simulink model "reaction_pendulum_MPC_swing_test"  (R2023b)
settings: Solver=FixedStepDiscrete  StartTime=0.0  StopTime=20  FixedStep=h  RelTol=1e-3  EnableMultiTasking=on
PreLoadFcn:
  | warning('off','MATLAB:dispatcher:InexactMatch');
InitFcn:
  | startup_sequence
StartFcn:
  | startup_sequence
model workspace (MAT data in the model file):
  square_freq = 0.5
values from neighbouring files (symbols this model uses):
  F = A22-L*A12    [Reduced_observer.m]
  G = A21-L*A11+F*L    [Reduced_observer.m]
  H = B2-L*B1    [Reduced_observer.m]
  K_LQR = lqr(A,B,Q,R)    [LQR_gain.m]
  L = 10    [LQR_gain.m]    (also in Reduced_observer.m = place(A22',A12',pole)')
  linearization_point = [0;0;0]    [startup_sequence.m]
  lp_deviation = [pi/9;0;0]    [startup_sequence.m]
undefined symbols (not defined in the file or in its folder): DiscIntNeverNeededParam, H_nlobs
libraries: mpclib x2
settings Model: ExtModeTrigDuration=100000  Creator=user  LastModifiedBy=india
settings DataIOCC: SaveFormat=Array  SignalLoggingSaveFormat=ModelDataLogs  SaveOutput=off  SignalLogging=off  DSMLogging=off  SaveTime=off  ReturnWorkspaceOutputs=off
settings OptimizationCC: ExpressionDepthLimit=2147483647  LifeSpan=inf
settings DebuggingCC: UnderspecifiedInitializationDetection=Classic  MergeDetectMultiDrivingBlocksExec=none  SolverPrmCheckMsg=warning  FcnCallInpInsideContextMsg=warning  UnconnectedInputMsg=warning  UnconnectedOutputMsg=warning  UnconnectedLineMsg=warning  StateNameClashWarn=warning  SFUnexpectedBacktrackingDiag=warning  SFNoUnconditionalDefaultTransitionDiag=warning  SFExecutionAtInitializationDiag=none  ArithmeticOperatorsInVariantConditions=warning
settings HardwareCC: ProdBitPerPointer=32  ProdBitPerSizeT=32  ProdBitPerPtrDiffT=32  ProdLargestAtomicFloat=None  ProdIntDivRoundTo=Undefined  ProdEndianess=Unspecified  ProdWordSize=32  ProdHWDeviceType=32-bit Generic
settings ModelReferenceCC: EnableRefExpFcnMdlSchedulingChecks=on  PropagateSignalLabelsOutOfModel=off
settings SFSimCC: SimUseLocalCustomCode=off  CustomCodeUndefinedFunction=UseInterfaceOnly
settings RTWCC: Description=rpend RTDAC/USB2 (Visual C/C++)  SystemTargetFile=rtcon_rpend_usb2.tlc  TemplateMakefile=rtcon_rpend_vc_usb2_x64.tmf  RTWUseLocalCustomCode=off  DLArmComputeVersion=19.05
settings CodeAppCC: StateflowObjectComments=on
settings STFCustomTargetCC: TargetLangStandard=C89/C90 (ANSI)  ModelReferenceCompliant=off  CombineOutputUpdateFcns=on  MatFileLogging=on  SystemTargetFile=rtcon_rpend_usb2.tlc
settings GRTTargetCC: TargetLangStandard=C89/C90 (ANSI)  ModelReferenceCompliant=off  ParMdlRefBuildCompliant=off  CompOptLevelCompliant=off  ConcurrentExecutionCompliant=off  CPPClassGenCompliant=off  UseToolchainInfoCompliant=off  ExtMode=on  ExtModeMexFile=rtcon_ext_comm
settings ConfigComp: CovMetricSettings=dw  CovSaveCumulativeToWorkspaceVar=on  CovSaveSingleToWorkspaceVar=on  CovExternalEMLEnable=off  CovSFcnEnable=off

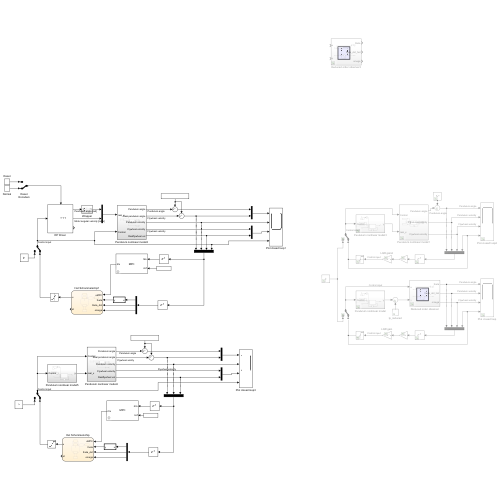
[thumbnail: Simulink's stored preview of the top-level diagram]
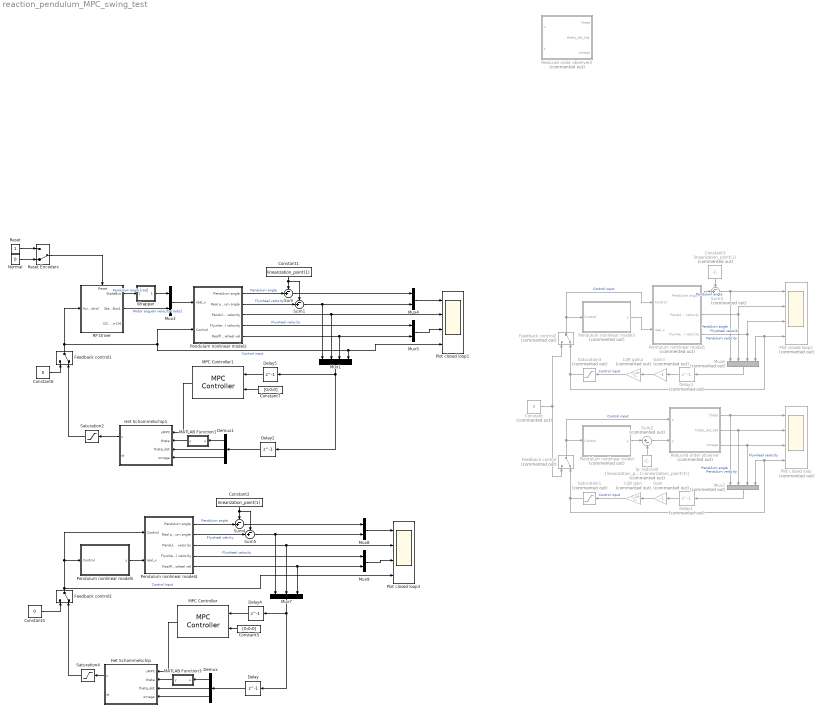
== system reaction_pendulum_MPC_swing_test ==
  Constant : Constant  Commented=on  Value=0
  Constant1 : Constant  Value=linearization_point(1)
  Constant2 : Constant  Value=linearization_point(1)
  Constant3 : Constant  Commented=on  Value=linearization_point(1)
  Constant4 : Constant  Value=0
  Constant5 : Constant  Value=[0;0;0]
  Constant6 : Constant  Value=0
  Constant7 : Constant  Value=[0;0;0]
  Delay{,2,4..5} (4 alike) : Delay  DelayLength=1
  Delay1 : Delay  Commented=on  DelayLength=1
  Delay3 : Delay  Commented=on  DelayLength=1
  Demux : Demux  Outputs=3
  Demux1 : Demux  Outputs=3
  Feedback control : ManualSwitch  Commented=on  CurrentSetting=0
  Feedback control1 : ManualSwitch  CurrentSetting=0
  Feedback control2 : ManualSwitch  Commented=on  CurrentSetting=0
  Feedback control3 : ManualSwitch  CurrentSetting=0
  Gain : Gain  Commented=on  Gain=-1
  Gain3 : Gain  Commented=on  Gain=-1
  Het Schommelschip : Stateflow chart  TreatAsAtomicUnit=on
      settings: PortSchema="{\"entries\":[{\"content\":{\"sides\":[{\"content\":{\"connectorIds\":[\"In3\",\"In1\",\"In2\",\"In4\"]},\"type\":\"ConnectorPlacement.EquallySpacedRectSide\",\"uuid\":\"5e0e74da-86d0-4b0f-97b8-22d473cf7e44\"},{\"content\":{\"connectorIds\":[\"Out1\",\"Out2\"],\"side\":\"RIGHT\"},\"type\":\"ConnectorPlacement.EquallySpacedRectSide\",\"uuid\":\"714d43ea-69d2-420e-91fb-73cc0bbad146\"},{\"content\":{\"side\":\"TOP\"},\"type\":\"ConnectorPlacement.EquallySpacedRectSide\",\"uuid\":\"53d3d334-5a38-461d-a9d2-49aa371a08e3\"}]},\"type\":\"ConnectorPlacement.EquallySpacedConnector\",\"uuid\":\"bed2510c-5cc6-4076-81b8-1d254a2b08c8\"}],\"packageUris\":[\"http://schema.mathworks.com/mf0/Connector/R2020b\"],\"version\":\"1.0\"}"
  Het Schommelschip1 : Stateflow chart  TreatAsAtomicUnit=on
      settings: PortSchema="{\"entries\":[{\"content\":{\"sides\":[{\"content\":{\"connectorIds\":[\"In3\",\"In1\",\"In2\",\"In4\"]},\"type\":\"ConnectorPlacement.EquallySpacedRectSide\",\"uuid\":\"5e0e74da-86d0-4b0f-97b8-22d473cf7e44\"},{\"content\":{\"connectorIds\":[\"Out1\",\"Out2\"],\"side\":\"RIGHT\"},\"type\":\"ConnectorPlacement.EquallySpacedRectSide\",\"uuid\":\"714d43ea-69d2-420e-91fb-73cc0bbad146\"},{\"content\":{\"side\":\"TOP\"},\"type\":\"ConnectorPlacement.EquallySpacedRectSide\",\"uuid\":\"53d3d334-5a38-461d-a9d2-49aa371a08e3\"}]},\"type\":\"ConnectorPlacement.EquallySpacedConnector\",\"uuid\":\"bed2510c-5cc6-4076-81b8-1d254a2b08c8\"}],\"packageUris\":[\"http://schema.mathworks.com/mf0/Connector/R2020b\"],\"version\":\"1.0\"}"
  LQR gain : Gain  Commented=on  Gain=K_LQR  Multiplication=Matrix(K*u)
  LQR gain2 : Gain  Commented=on  Gain=K_LQR  Multiplication=Matrix(K*u)
  MATLAB Function1 : MATLAB Function  TreatAsAtomicUnit=on
  MATLAB Function3 : MATLAB Function  TreatAsAtomicUnit=on
  MPC Controller : mpclib/MPC Controller  SCDEnableBlockLinearizationSpecification=on  mpcobj=mpc_controller  is_multiple=0  enable_value=0  return_u0=off  updateMPCinCallerWorkspace=on  md_inport=off  mv_inport=off  uref_inport=off  return_cost=off  return_mvseq=off  return_qpstatus=off  return_xseq=off  return_state=off  return_ovseq=off  state_inport=off  umin_inport=off  umax_inport=off  ymin_inport=off  ymax_inport=off  cc_inport=off  ywt_inport=off  uwt_inport=off  duwt_inport=off  rhoeps_inport=off  pm_inport=off  MaximumP=10  HorizonChoice=FixedHorizon  n_ts=0.01  n_p=20  n_mv=1  n_md=0  n_ud=0  n_mo=3  n_uo=0  BlockDataType=double  SampleTimeInherited=off  switch_inport=off
  MPC Controller1 : mpclib/MPC Controller  SCDEnableBlockLinearizationSpecification=on  mpcobj=mpc_controller  is_multiple=0  enable_value=0  return_u0=off  updateMPCinCallerWorkspace=on  md_inport=off  mv_inport=off  uref_inport=off  return_cost=off  return_mvseq=off  return_qpstatus=off  return_xseq=off  return_state=off  return_ovseq=off  state_inport=off  umin_inport=off  umax_inport=off  ymin_inport=off  ymax_inport=off  cc_inport=off  ywt_inport=off  uwt_inport=off  duwt_inport=off  rhoeps_inport=off  pm_inport=off  MaximumP=10  HorizonChoice=FixedHorizon  n_ts=0.01  n_p=20  n_mv=1  n_md=0  n_ud=0  n_mo=3  n_uo=0  BlockDataType=double  SampleTimeInherited=off  switch_inport=off
  Mux1 : Mux
  Mux2 : Mux  Commented=on
  Mux{3..5,8..9} (5 alike) : Mux  Inputs=2
  Mux6 : Mux  Commented=on
  Mux7 : Mux  Inputs=3
  Normal : Constant  Value=0
  Pendulum nonlinear model : Subsystem  Commented=on
  Pendulum nonlinear model1 : Subsystem  Commented=on
  Pendulum nonlinear model2 : Subsystem
  Pendulum nonlinear model3 : Subsystem  Commented=on
  Pendulum nonlinear model4 : Subsystem
  Pendulum nonlinear model5 : Subsystem
  Plot closed loop : Scope  Commented=on  NumInputPorts=4
  Plot closed loop1 : Scope  NumInputPorts=4
  Plot closed loop2 : Scope  Commented=on  NumInputPorts=4
  Plot closed loop3 : Scope  NumInputPorts=4
  RP Driver : Subsystem
      settings: PortSchema="{\"entries\":[{\"content\":{\"sides\":[{\"content\":{\"connectorIds\":[\"In1\"]},\"type\":\"ConnectorPlacement.EquallySpacedRectSide\",\"uuid\":\"28df0a7f-6242-4d39-ac1c-ff3ee0c6a4e1\"},{\"content\":{\"connectorIds\":[\"Out1\",\"Out2\",\"Out3\"],\"side\":\"RIGHT\"},\"type\":\"ConnectorPlacement.EquallySpacedRectSide\",\"uuid\":\"435de4ce-8687-493c-bad7-12ebb99ee6db\"},{\"content\":{\"connectorIds\":[\"In2\"],\"side\":\"TOP\"},\"type\":\"ConnectorPlacement.EquallySpacedRectSide\",\"uuid\":\"946ce8c1-4b6f-49e8-9b13-de0bfa90dc27\"},{\"content\":{\"side\":\"BOTTOM\"},\"type\":\"ConnectorPlacement.EquallySpacedRectSide\",\"uuid\":\"2521f2e0-71e2-448f-85b3-c4d5eb7ca065\"}]},\"type\":\"ConnectorPlacement.EquallySpacedConnector\",\"uuid\":\"0b989423-35e3-4087-b06d-cef0c97f9c21\"}],\"packageUris\":[\"http://schema.mathworks.com/mf0/Connector/R2020b\"],\"version\":\"1.0\"}"
      mask Display: image(imread('rwp.JPG'))
  Reduced order observer : Subsystem  Commented=on
  Reduced order observer2 : Subsystem  Commented=on
  Reset : Constant
  Reset Encoders : ManualSwitch  CurrentSetting=0
  Saturation1 : Saturate  Commented=on  UpperLimit=1  LowerLimit=-1
  Saturation2 : Saturate  UpperLimit=1  LowerLimit=-1
  Saturation3 : Saturate  Commented=on  UpperLimit=1  LowerLimit=-1
  Saturation4 : Saturate  UpperLimit=1  LowerLimit=-1
  Sum{,1,4..5} (4 alike) : Sum  Inputs=-+|
  Sum2 : Sum  Commented=on  Inputs=|+-
  Sum3 : Sum  Commented=on  Inputs=-+|
  Wrapper : Subsystem
  lp_reduced : Constant  Commented=on  Value=[linearization_point(1);linearization_point(3)]
  wires:
  Normal/1 -> Reset Encoders/2
  Reset/1 -> Reset Encoders/1
  Reset Encoders/1 -> RP Driver/2(Reset)
  RP Driver/1(StateBus) -> Wrapper/1(In1)  "Pendulum angle [rad]"
  Feedback control/1 -> Reduced order observer/1(u), Pendulum nonlinear model/1(Control)  "Control input"
  LQR gain/1 -> Saturation1/1  "Control input"
  Gain/1 -> LQR gain/1
  Delay1/1 -> Gain/1
  Reduced order observer/2(theta_dot_hat) -> Plot closed loop/2, Mux2/2  "Pendulum velocity"
  Sum2/1 -> Reduced order observer/2(y)
  lp_reduced/1 -> Sum2/2
  Pendulum nonlinear model/1(y) -> Sum2/1
  Reduced order observer/1(theta) -> Plot closed loop/1, Mux2/1  "Pendulum angle"
  Reduced order observer/3(omega) -> Plot closed loop/3, Mux2/3  "Flywheel velocity"
  Mux2/1 -> Delay1/1
  Feedback control1/1 -> Pendulum nonlinear model2/2(Control), Mux1/4, Plot closed loop1/4, RP Driver/1(Azimuth Control)  "Control input"
  Saturation1/1 -> Plot closed loop/4, Mux2/4, Feedback control/2
  Constant1/1 -> Sum1/1, Sum/1
  Wrapper/1(Out1) -> Mux3/1
  Mux4/1 -> Plot closed loop1/1
  Mux5/1 -> Plot closed loop1/3
  Sum1/1 -> Mux4/2, Mux1/1
  Pendulum nonlinear model1/1(Pendulum angle) -> Sum3/2  "Pendulum angle"
  Constant3/1 -> Sum3/1
  Saturation3/1 -> Plot closed loop2/4, Mux6/4, Feedback control2/2
  Pendulum nonlinear model3/1(y) -> Pendulum nonlinear model1/2(real_x)
  Sum3/1 -> Plot closed loop2/1, Mux6/1  "Pendulum angle"
  Gain3/1 -> LQR gain2/1
  Pendulum nonlinear model1/2(Pendulum velocity) -> Plot closed loop2/2, Mux6/2  "Pendulum velocity"
  LQR gain2/1 -> Saturation3/1  "Control input"
  Pendulum nonlinear model1/3(Flywheel velocity) -> Plot closed loop2/3, Mux6/3  "Flywheel velocity"
  Mux6/1 -> Delay3/1
  Delay3/1 -> Gain3/1
  Feedback control2/1 -> Pendulum nonlinear model3/1(Control), Pendulum nonlinear model1/1(Control)  "Control input"
  Constant/1 -> Feedback control/1, Feedback control2/1
  Feedback control3/1 -> Pendulum nonlinear model4/1(Control), Pendulum nonlinear model5/1(Control), Plot closed loop3/4  "Control input"
  Pendulum nonlinear model5/1(y) -> Pendulum nonlinear model4/2(real_x)
  Constant4/1 -> Feedback control3/1
  Constant6/1 -> Feedback control1/1
  RP Driver/2(StateBus1) -> Mux3/2  "Motor angular velocity [rad/s]"
  Sum/1 -> Mux4/1
  Sum4/1 -> Mux8/1
  Pendulum nonlinear model4/4(Flywheel velocity) -> Mux9/1  "Flywheel velocity"
  Pendulum nonlinear model4/5(Realflywheel vel) -> Mux7/3, Mux9/2
  Mux9/1 -> Plot closed loop3/3
  Mux8/1 -> Plot closed loop3/1
  Sum5/1 -> Mux8/2, Mux7/1
  Pendulum nonlinear model4/1(Pendulum angle) -> Sum4/2  "Pendulum angle"
  Constant2/1 -> Sum5/1, Sum4/1
  Mux7/1 -> Delay/1, Delay4/1
  Pendulum nonlinear model4/3(Pendulum velocity) -> Mux7/2, Plot closed loop3/2
  Pendulum nonlinear model4/2(Real pendulum angle) -> Sum5/2  "Flywheel velcity"
  Pendulum nonlinear model2/1(Pendulum angle) -> Sum/2  "Pendulum angle"
  Pendulum nonlinear model2/2(Real pendulum angle) -> Sum1/2  "Flywheel velocity"
  Pendulum nonlinear model2/3(Pendulum velocity) -> Mux1/2, Plot closed loop1/2
  Pendulum nonlinear model2/4(Flywheel velocity) -> Mux5/1  "Flywheel velocity"
  Pendulum nonlinear model2/5(Realflywheel vel) -> Mux5/2, Mux1/3
  Mux3/1 -> Pendulum nonlinear model2/1(real_x)
  Delay4/1 -> MPC Controller/1
  Demux/3 -> Het Schommelschip/4(omega)
  Demux/1 -> MATLAB Function3/1(u)
  MATLAB Function3/1(y) -> Het Schommelschip/1(theta)
  Demux/2 -> Het Schommelschip/2(theta_dot)
  Het Schommelschip/1(u) -> Saturation4/1
  MPC Controller/1 -> Het Schommelschip/3(uMPC)
  Constant5/1 -> MPC Controller/2
  Delay/1 -> Demux/1
  Saturation4/1 -> Feedback control3/2
  Saturation2/1 -> Feedback control1/2
  Demux1/2 -> Het Schommelschip1/2(theta_dot)
  Delay2/1 -> Demux1/1
  Demux1/1 -> MATLAB Function1/1(u)
  Constant7/1 -> MPC Controller1/2
  Demux1/3 -> Het Schommelschip1/4(omega)
  MPC Controller1/1 -> Het Schommelschip1/3(uMPC)
  MATLAB Function1/1(y) -> Het Schommelschip1/1(theta)
  Delay5/1 -> MPC Controller1/1
  Het Schommelschip1/1(u) -> Saturation2/1
  Mux1/1 -> Delay5/1, Delay2/1

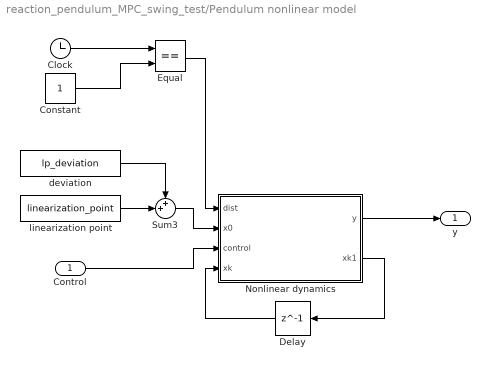
== system reaction_pendulum_MPC_swing_test/Pendulum nonlinear model ==
  Control : Inport
  Clock : Clock
  Constant : Constant
  Delay : Delay  DelayLength=1
  Equal : RelationalOperator  Operator===  OutDataTypeStr=boolean  RndMeth=Simplest  InputSameDT=off
  Nonlinear dynamics : MATLAB Function  TreatAsAtomicUnit=on
  Sum3 : Sum  Inputs=++|
  deviation : Constant  Value=lp_deviation
  linearization point : Constant  Value=linearization_point
  y : Outport
  wires:
  Delay/1 -> Nonlinear dynamics/4(xk)
  Sum3/1 -> Nonlinear dynamics/2(x0)
  Control/1 -> Nonlinear dynamics/3(control)
  Nonlinear dynamics/2(xk1) -> Delay/1
  Nonlinear dynamics/1(y) -> y/1
  deviation/1 -> Sum3/1
  linearization point/1 -> Sum3/2
  Constant/1 -> Equal/2
  Equal/1 -> Nonlinear dynamics/1(dist)
  Clock/1 -> Equal/1

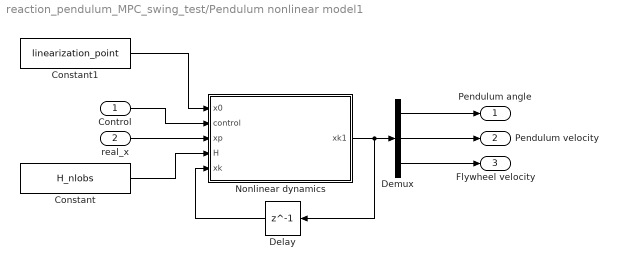
== system reaction_pendulum_MPC_swing_test/Pendulum nonlinear model1 ==
  Control : Inport
  real_x : Inport  Port=2
  Constant : Constant  Value=H_nlobs
  Constant1 : Constant  Value=linearization_point
  Delay : Delay  DelayLength=1
  Demux : Demux  Outputs=3
  Nonlinear dynamics : MATLAB Function  TreatAsAtomicUnit=on
  Pendulum angle : Outport
  Pendulum velocity : Outport  Port=2
  Flywheel velocity : Outport  Port=3
  wires:
  Delay/1 -> Nonlinear dynamics/5(xk)
  Control/1 -> Nonlinear dynamics/2(control)
  Nonlinear dynamics/1(xk1) -> Demux/1, Delay/1
  real_x/1 -> Nonlinear dynamics/3(xp)
  Constant/1 -> Nonlinear dynamics/4(H)
  Constant1/1 -> Nonlinear dynamics/1(x0)
  Demux/2 -> Pendulum velocity/1
  Demux/1 -> Pendulum angle/1
  Demux/3 -> Flywheel velocity/1

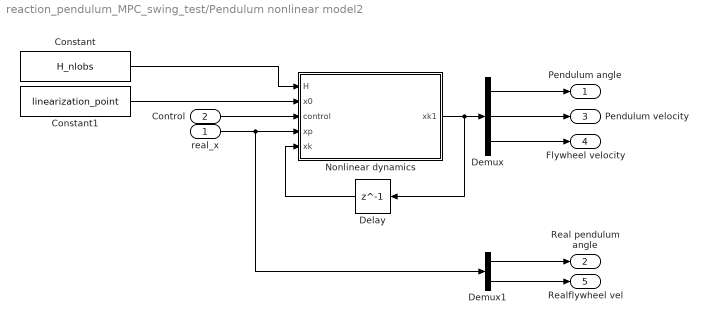
== system reaction_pendulum_MPC_swing_test/Pendulum nonlinear model2 ==
  real_x : Inport
  Control : Inport  Port=2
  Constant : Constant  Value=H_nlobs
  Constant1 : Constant  Value=linearization_point
  Delay : Delay  DelayLength=1
  Demux : Demux  Outputs=3
  Demux1 : Demux  Outputs=2
  Nonlinear dynamics : MATLAB Function  TreatAsAtomicUnit=on
  Pendulum angle : Outport
  Real pendulum angle : Outport  Port=2
  Pendulum velocity : Outport  Port=3
  Flywheel velocity : Outport  Port=4
  Realflywheel vel : Outport  Port=5
  wires:
  Delay/1 -> Nonlinear dynamics/5(xk)
  Control/1 -> Nonlinear dynamics/3(control)
  Nonlinear dynamics/1(xk1) -> Demux/1, Delay/1
  real_x/1 -> Demux1/1, Nonlinear dynamics/4(xp)
  Constant/1 -> Nonlinear dynamics/1(H)
  Constant1/1 -> Nonlinear dynamics/2(x0)
  Demux/2 -> Pendulum velocity/1
  Demux/1 -> Pendulum angle/1
  Demux/3 -> Flywheel velocity/1
  Demux1/1 -> Real pendulum angle/1
  Demux1/2 -> Realflywheel vel/1

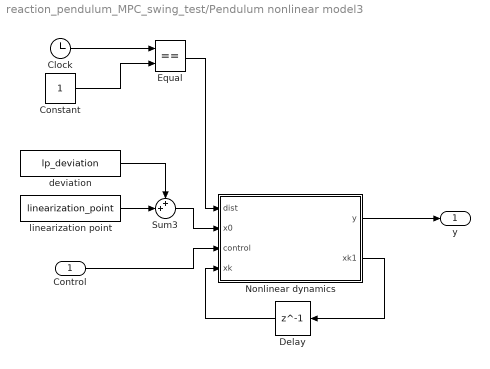
== system reaction_pendulum_MPC_swing_test/Pendulum nonlinear model3 ==
  Control : Inport
  Clock : Clock
  Constant : Constant
  Delay : Delay  DelayLength=1
  Equal : RelationalOperator  Operator===  OutDataTypeStr=boolean  RndMeth=Simplest  InputSameDT=off
  Nonlinear dynamics : MATLAB Function  TreatAsAtomicUnit=on
  Sum3 : Sum  Inputs=++|
  deviation : Constant  Value=lp_deviation
  linearization point : Constant  Value=linearization_point
  y : Outport
  wires:
  Delay/1 -> Nonlinear dynamics/4(xk)
  Sum3/1 -> Nonlinear dynamics/2(x0)
  Control/1 -> Nonlinear dynamics/3(control)
  Nonlinear dynamics/2(xk1) -> Delay/1
  Nonlinear dynamics/1(y) -> y/1
  deviation/1 -> Sum3/1
  linearization point/1 -> Sum3/2
  Clock/1 -> Equal/1
  Constant/1 -> Equal/2
  Equal/1 -> Nonlinear dynamics/1(dist)

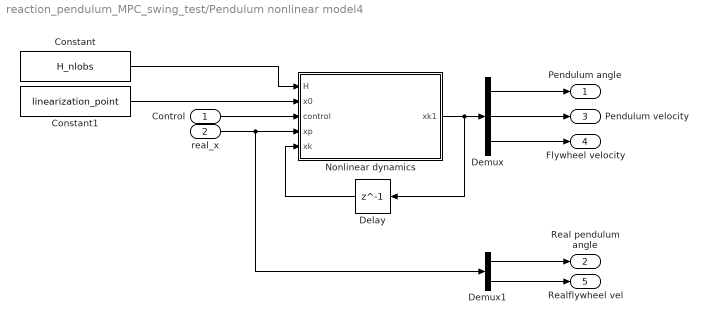
== system reaction_pendulum_MPC_swing_test/Pendulum nonlinear model4 ==
  Control : Inport
  real_x : Inport  Port=2
  Constant : Constant  Value=H_nlobs
  Constant1 : Constant  Value=linearization_point
  Delay : Delay  DelayLength=1
  Demux : Demux  Outputs=3
  Demux1 : Demux  Outputs=2
  Nonlinear dynamics : MATLAB Function  TreatAsAtomicUnit=on
  Pendulum angle : Outport
  Real pendulum angle : Outport  Port=2
  Pendulum velocity : Outport  Port=3
  Flywheel velocity : Outport  Port=4
  Realflywheel vel : Outport  Port=5
  wires:
  Delay/1 -> Nonlinear dynamics/5(xk)
  Control/1 -> Nonlinear dynamics/3(control)
  Nonlinear dynamics/1(xk1) -> Demux/1, Delay/1
  real_x/1 -> Demux1/1, Nonlinear dynamics/4(xp)
  Constant/1 -> Nonlinear dynamics/1(H)
  Constant1/1 -> Nonlinear dynamics/2(x0)
  Demux/2 -> Pendulum velocity/1
  Demux/1 -> Pendulum angle/1
  Demux/3 -> Flywheel velocity/1
  Demux1/1 -> Real pendulum angle/1
  Demux1/2 -> Realflywheel vel/1

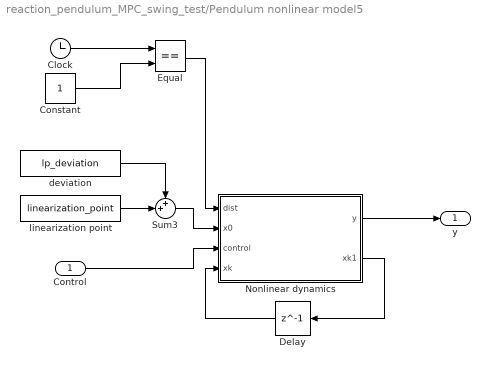
== system reaction_pendulum_MPC_swing_test/Pendulum nonlinear model5 ==
  Control : Inport
  Clock : Clock
  Constant : Constant
  Delay : Delay  DelayLength=1
  Equal : RelationalOperator  Operator===  OutDataTypeStr=boolean  RndMeth=Simplest  InputSameDT=off
  Nonlinear dynamics : MATLAB Function  TreatAsAtomicUnit=on
  Sum3 : Sum  Inputs=++|
  deviation : Constant  Value=lp_deviation
  linearization point : Constant  Value=linearization_point
  y : Outport
  wires:
  Delay/1 -> Nonlinear dynamics/4(xk)
  Sum3/1 -> Nonlinear dynamics/2(x0)
  Control/1 -> Nonlinear dynamics/3(control)
  Nonlinear dynamics/2(xk1) -> Delay/1
  Nonlinear dynamics/1(y) -> y/1
  deviation/1 -> Sum3/1
  linearization point/1 -> Sum3/2
  Clock/1 -> Equal/1
  Constant/1 -> Equal/2
  Equal/1 -> Nonlinear dynamics/1(dist)

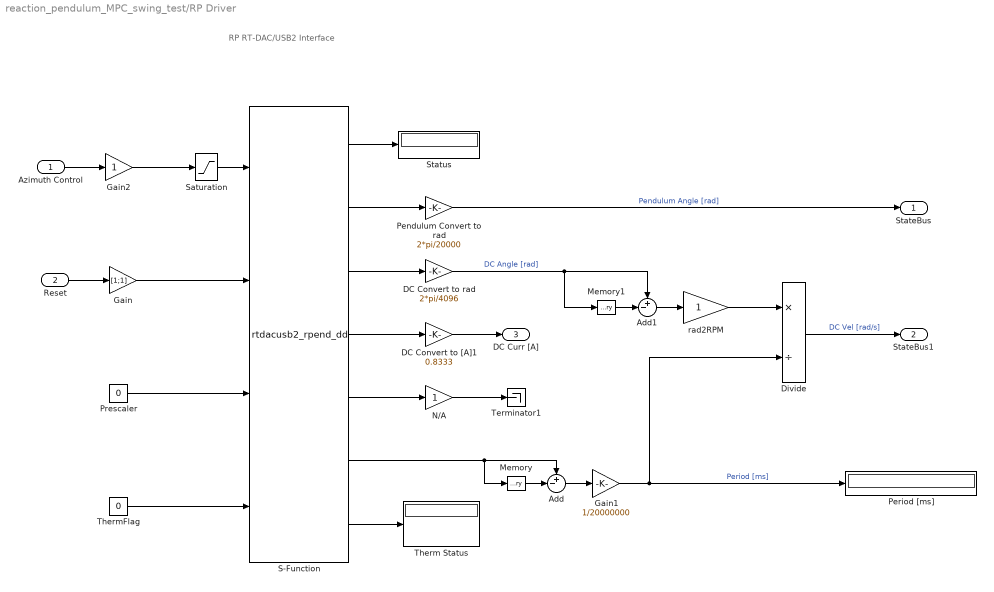
== system reaction_pendulum_MPC_swing_test/RP Driver ==
  note: RP RT-DAC/USB2
      | Interface
  Azimuth Control : Inport
  Reset : Inport  Port=2
  Add : Sum  Inputs=+-|
  Add1 : Sum  Inputs=+-|
  DC Convert to [A]1 : Gain  Gain=0.8333  SaturateOnIntegerOverflow=on  OutDataTypeStr=Inherit: Same as input  ParamDataTypeStr=Inherit: Same as input
  DC Convert to rad : Gain  Gain=2*pi/4096  SaturateOnIntegerOverflow=on  OutDataTypeStr=Inherit: Same as input  ParamDataTypeStr=Inherit: Same as input
  Divide : Product  Inputs=*/
  Gain : Gain  Gain=[1;1]
  Gain1 : Gain  Gain=1/20000000
  Gain2 : Gain
  Memory : Memory
  Memory1 : Memory
  N/A : Gain  SaturateOnIntegerOverflow=on  OutDataTypeStr=Inherit: Same as input  ParamDataTypeStr=Inherit: Same as input
  Pendulum Convert to rad : Gain  Gain=2*pi/20000  SaturateOnIntegerOverflow=on  OutDataTypeStr=Inherit: Same as input  ParamDataTypeStr=Inherit: Same as input
  Period [ms] : Display
  Prescaler : Constant  Value=0
  S-Function : S-Function  FunctionName=rtdacusb2_rpend_dd  Parameters=1, h  SFunctionDeploymentMode=off  EnableBusSupport=off
  Saturation : Saturate  UpperLimit=1  LowerLimit=-1
  Status : Display
  Terminator1 : Terminator
  Therm Status : Display
  ThermFlag : Constant  Value=0
  rad2RPM : Gain  SaturateOnIntegerOverflow=on  OutDataTypeStr=Inherit: Same as input  ParamDataTypeStr=Inherit: Same as input
  StateBus : Outport  VectorParamsAs1DForOutWhenUnconnected=off
  StateBus1 : Outport  Port=2  VectorParamsAs1DForOutWhenUnconnected=off
  DC Curr [A] : Outport  Port=3  VectorParamsAs1DForOutWhenUnconnected=off
  wires:
  S-Function/7 -> Therm Status/1
  S-Function/5 -> N/A/1
  S-Function/4 -> DC Convert to [A]1/1
  ThermFlag/1 -> S-Function/4
  Prescaler/1 -> S-Function/3
  Gain/1 -> S-Function/2
  DC Convert to [A]1/1 -> DC Curr [A]/1
  Divide/1 -> StateBus1/1  "DC Vel [rad/s]"
  rad2RPM/1 -> Divide/1
  Add1/1 -> rad2RPM/1
  Memory1/1 -> Add1/2
  N/A/1 -> Terminator1/1
  S-Function/6 -> Add/1, Memory/1
  Gain2/1 -> Saturation/1
  Gain1/1 -> Period [ms]/1, Divide/2  "Period [ms]"
  Add/1 -> Gain1/1
  Memory/1 -> Add/2
  DC Convert to rad/1 -> Add1/1, Memory1/1  "DC Angle [rad]"
  S-Function/3 -> DC Convert to rad/1
  Pendulum Convert to rad/1 -> StateBus/1  "Pendulum Angle [rad]"
  S-Function/2 -> Pendulum Convert to rad/1
  S-Function/1 -> Status/1
  Saturation/1 -> S-Function/1
  Reset/1 -> Gain/1
  Azimuth Control/1 -> Gain2/1

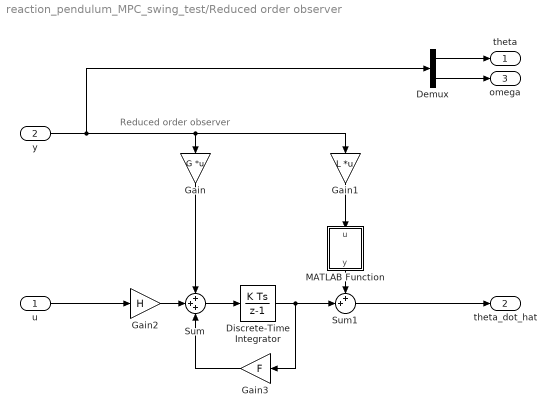
== system reaction_pendulum_MPC_swing_test/Reduced order observer ==
  note: Reduced order observer
  u : Inport
  y : Inport  Port=2
  Demux : Demux  Outputs=2
  Discrete-Time Integrator : DiscreteIntegrator  SampleTime=-1  ICPrevOutput=DiscIntNeverNeededParam  ICPrevScaledInput=DiscIntNeverNeededParam
  Gain : Gain  Gain=G  Multiplication=Matrix(K*u)
  Gain1 : Gain  Gain=L  Multiplication=Matrix(K*u)
  Gain2 : Gain  Gain=H
  Gain3 : Gain  Gain=F
  MATLAB Function : MATLAB Function  TreatAsAtomicUnit=on
  Sum : Sum  Inputs=+++
  Sum1 : Sum  Inputs=++|
  theta : Outport
  theta_dot_hat : Outport  Port=2
  omega : Outport  Port=3
  wires:
  u/1 -> Gain2/1
  Gain2/1 -> Sum/2
  Gain/1 -> Sum/1
  Sum/1 -> Discrete-Time Integrator/1
  Discrete-Time Integrator/1 -> Gain3/1, Sum1/2
  Gain3/1 -> Sum/3
  Sum1/1 -> theta_dot_hat/1
  y/1 -> Gain1/1, Gain/1, Demux/1
  Demux/1 -> theta/1
  Demux/2 -> omega/1
  Gain1/1 -> MATLAB Function/1(u)
  MATLAB Function/1(y) -> Sum1/1

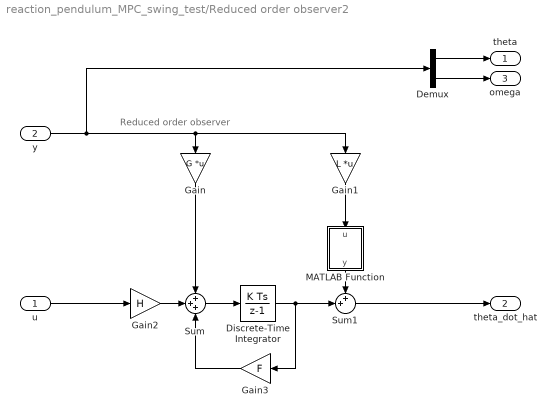
== system reaction_pendulum_MPC_swing_test/Reduced order observer2 ==
  note: Reduced order observer
  u : Inport
  y : Inport  Port=2
  Demux : Demux  Outputs=2
  Discrete-Time Integrator : DiscreteIntegrator  SampleTime=-1  ICPrevOutput=DiscIntNeverNeededParam  ICPrevScaledInput=DiscIntNeverNeededParam
  Gain : Gain  Gain=G  Multiplication=Matrix(K*u)
  Gain1 : Gain  Gain=L  Multiplication=Matrix(K*u)
  Gain2 : Gain  Gain=H
  Gain3 : Gain  Gain=F
  MATLAB Function : MATLAB Function  TreatAsAtomicUnit=on
  Sum : Sum  Inputs=+++
  Sum1 : Sum  Inputs=++|
  theta : Outport
  theta_dot_hat : Outport  Port=2
  omega : Outport  Port=3
  wires:
  u/1 -> Gain2/1
  Gain2/1 -> Sum/2
  Gain/1 -> Sum/1
  Sum/1 -> Discrete-Time Integrator/1
  Discrete-Time Integrator/1 -> Gain3/1, Sum1/2
  Gain3/1 -> Sum/3
  Sum1/1 -> theta_dot_hat/1
  y/1 -> Gain1/1, Gain/1, Demux/1
  Demux/1 -> theta/1
  Demux/2 -> omega/1
  Gain1/1 -> MATLAB Function/1(u)
  MATLAB Function/1(y) -> Sum1/1

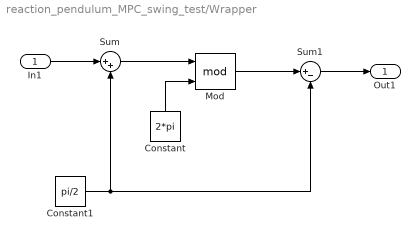
== system reaction_pendulum_MPC_swing_test/Wrapper ==
  In1 : Inport
  Constant : Constant  Value=2*pi
  Constant1 : Constant  Value=pi/2
  Mod : Math  Operator=mod
  Sum : Sum  Inputs=|++
  Sum1 : Sum  Inputs=|+-
  Out1 : Outport
  wires:
  Constant/1 -> Mod/2
  Mod/1 -> Sum1/1
  Sum1/1 -> Out1/1
  In1/1 -> Sum/1
  Sum/1 -> Mod/1
  Constant1/1 -> Sum1/2, Sum/2

== matlab function reaction_pendulum_MPC_swing_test/Reduced order observer2/MATLAB Function ==
  data: u input; y output
function y = fcn(u)
    persistent obs_init
    y=u;
    if isempty(obs_init)
        y=0;
        obs_init = true;
    end
end

== matlab function reaction_pendulum_MPC_swing_test/Pendulum nonlinear model3/Nonlinear dynamics ==
  data: dist input; x0 input; y output; control input; xk input size=[3,1]; xk1 output size=[3,1]; h parameter
function [y, xk1] = nlrk4(dist, x0, control, xk, h)
    persistent initialized

    if isempty(initialized)
        xk = x0;
        initialized = true;
    end

    function dx = nlf(t,x,u)
    
        % Define constants
        K1 = 10.6608;
        K2 = 0.0487;
        K3 = 0.1031;
        K4 = 404.3827;
        K5 = 0.9442;
        K6 = 1.7125;
        K_tau = 0.0107;
        
        % System equations
        theta = x(1);
        theta_dot = x(2);
        omega = x(3);
        theta_ddot = -K1*sin(theta)-K2*theta_dot-K3*sign(theta_dot)-K_tau*(K4*u-K5*omega-K6*sign(omega));
        omega_dot = K4*u-K5*omega-K6*sign(omega);
        dx = [theta_dot; theta_ddot; omega_dot];
    end

    % Executes one timestep of the RK4 algorithm
    k1 = nlf(0, xk, control);
    k2 = nlf(0 + h/2, xk + h/2*k1, control);
    k3 = nlf(0 + h/2, xk + h/2*k2, control);
    k4 = nlf(0 + h, xk + h*k3, control);
    xk1 = xk + h/6*(k1 + 2*k2 + 2*k3 + k4);
    
    if dist
        xk1(1)=pi+deg2rad(5);
        xk(1) =pi+deg2rad(5);
    end

    % % Forward Euler
    % xk1 = xk + h*nlf(0, xk, control);
    % Take out states of interest
    y = [xk(1); xk(3)];
end

== matlab function reaction_pendulum_MPC_swing_test/Pendulum nonlinear model4/Nonlinear dynamics ==
  data: H input; x0 input; control input; xp input; xk input size=[3,1]; xk1 output size=[3,1]; h parameter
function xk1   = nlrk4(H, x0, control, xp, xk, h)
    persistent initialized

    if isempty(initialized)
        xk1 = x0;
        theta_dd = 0;
        initialized = true;
        return;
    end

    function dx = nlf(t,x,u,xp,H)
        C = [1,0,0;0,0,1];

        % Define constants
        K1 = 10.6608;
        K2 = 0.0487;
        K3 = 0.1031;
        K4 = 404.3827;
        K5 = 0.9442;
        K6 = 1.7125;
        K_tau = 0.0107;
        
        % System equations
        theta = x(1);
        theta_dot = x(2);
        omega = x(3);
        theta_ddot = -K1*sin(theta)-K2*theta_dot-K3*sign(theta_dot)-K_tau*(K4*u-K5*omega-K6*sign(omega));
        omega_dot = K4*u-K5*omega-K6*sign(omega);
        delta = xp-C*x;
        Linear_term = H*(delta);
        NL_term = [theta_dot; theta_ddot; omega_dot] ;
        dx = NL_term + Linear_term;
    end

    function theta_ddot = theta_ddd(t,x,u,xp,H)
        C = [1,0,0;0,0,1];

        % Define constants
        K1 = 10.6608;
        K2 = 0.0487;
        K3 = 0.1031;
        K4 = 404.3827;
        K5 = 0.9442;
        K6 = 1.7125;
        K_tau = 0.0107;
        
        % System equations
        theta = x(1);
        theta_dot = x(2);
        omega = x(3);
        theta_ddot = -K1*sin(theta)-K2*theta_dot-K3*sign(theta_dot)-K_tau*(K4*u-K5*omega-K6*sign(omega));
    end

    theta_dd = theta_ddd(0, xk, control, xp, H);

    % Executes one timestep of the RK4 algorithm
    k1 = nlf(0, xk, control, xp, H);
    k2 = nlf(0 + h/2, xk + h/2*k1, control, xp + h/2*k1([1,3]), H);
    k3 = nlf(0 + h/2, xk + h/2*k2, control, xp + h/2*k2([1,3]), H);
    k4 = nlf(0 + h, xk + h*k3, control, xp + h*k3([1,3]), H);
    xk1 = xk + h/6*(k1 + 2*k2 + 2*k3 + k4);

    % % Forward Euler
    % xk1 = xk + h*nlf(0, xk, control);
    % Take out states of interest
    % y = [xk(1); xk(3)];
end

== matlab function reaction_pendulum_MPC_swing_test/Pendulum nonlinear model5/Nonlinear dynamics ==
  data: dist input; x0 input; y output; control input; xk input size=[3,1]; xk1 output size=[3,1]; h parameter
function [y, xk1] = nlrk4(dist, x0, control, xk, h)
    persistent initialized

    if isempty(initialized)
        xk = x0;
        initialized = true;
    end

    function dx = nlf(t,x,u)
    
        % Define constants
        K1 = 10.6608;
        K2 = 0.0487;
        K3 = 0.1031;
        K4 = 404.3827;
        K5 = 0.9442;
        K6 = 1.7125;
        K_tau = 0.0107;
        
        % System equations
        theta = x(1);
        theta_dot = x(2);
        omega = x(3);
        theta_ddot = -K1*sin(theta)-K2*theta_dot-K3*sign(theta_dot)-K_tau*(K4*u-K5*omega-K6*sign(omega));
        omega_dot = K4*u-K5*omega-K6*sign(omega);
        dx = [theta_dot; theta_ddot; omega_dot];
    end

    % Executes one timestep of the RK4 algorithm
    k1 = nlf(0, xk, control);
    k2 = nlf(0 + h/2, xk + h/2*k1, control);
    k3 = nlf(0 + h/2, xk + h/2*k2, control);
    k4 = nlf(0 + h, xk + h*k3, control);
    xk1 = xk + h/6*(k1 + 2*k2 + 2*k3 + k4);

    % if dist
    %     xk1(1)=pi/9;
    %     xk(1) = pi/9;
    % end

    % % Forward Euler
    % xk1 = xk + h*nlf(0, xk, control);
    % Take out states of interest
    y = [xk(1); xk(3)];
end

== stateflow chart reaction_pendulum_MPC_swing_test/Het Schommelschip1 ==
  state Swing_up
    u=-ku*sign(theta_dot);
    st = -0.1;
  state Nothing
    u=0;
    st = 0;
  state Slow_down
    u=kp*sign(theta_dot);
    st = 0.1;
  state Stabilizing
    u=uMPC;
    st=0.4;
  state Flywheel_limit
    u=0;
  Nothing -> Swing_up [order 1] : [abs(theta)>wheel]
  Swing_up -> Nothing : [abs(theta)<wheel]
  Nothing -> Slow_down [order 3] : [abs(theta)<pi/2 && abs(theta_dot)>vmax]
  Slow_down -> Nothing : [abs(theta_dot)<vmax]
  Nothing -> Stabilizing [order 2] : [abs(theta) < delta]
  Stabilizing -> Nothing [order 1] : [abs(theta) > delta]
  (default) -> Nothing
  Flywheel_limit -> Stabilizing : [abs(omega)<200]
  Stabilizing -> Flywheel_limit [order 2] : [abs(omega)>250]
  data: theta input; theta_dot input; u output; ku local =0.75; kp local =1; delta local =deg2rad(20); uMPC input; vmax local =5; wheel local =3*pi/4; st output; omega input

== matlab function reaction_pendulum_MPC_swing_test/MATLAB Function1 ==
  data: u input; y output
function y = fcn(u)

y = mod(u,2*pi)-pi;

end

== stateflow chart reaction_pendulum_MPC_swing_test/Het Schommelschip ==
  state Swing_up
    u=-ku*sign(theta_dot);
    st = -0.1;
  state Nothing
    u=0;
    st = 0;
  state Slow_down
    u=kp*sign(theta_dot);
    st = 0.1;
  state Stabilizing
    u=uMPC;
    st=0.4;
  state Flywheel_limit
    u=0;
  Nothing -> Swing_up [order 1] : [abs(theta)>wheel]
  Swing_up -> Nothing : [abs(theta)<wheel]
  Nothing -> Slow_down [order 3] : [abs(theta)<pi/2 && abs(theta_dot)>vmax]
  Slow_down -> Nothing : [abs(theta_dot)<vmax]
  Nothing -> Stabilizing [order 2] : [abs(theta) < delta]
  Stabilizing -> Nothing [order 1] : [abs(theta) > delta]
  (default) -> Nothing
  Flywheel_limit -> Stabilizing : [abs(omega)<200]
  Stabilizing -> Flywheel_limit [order 2] : [abs(omega)>250]
  data: theta input; theta_dot input; u output; ku local =0.75; kp local =1; delta local =deg2rad(20); uMPC input; vmax local =5; wheel local =3*pi/4; st output; omega input

== matlab function reaction_pendulum_MPC_swing_test/MATLAB Function3 ==
  data: u input; y output
function y = fcn(u)

y = mod(u,2*pi)-pi;

end

== matlab function reaction_pendulum_MPC_swing_test/Reduced order observer/MATLAB Function ==
  data: u input; y output
function y = fcn(u)
    persistent obs_init
    y=u;
    if isempty(obs_init)
        y=0;
        obs_init = true;
    end
end

== matlab function reaction_pendulum_MPC_swing_test/Pendulum nonlinear model/Nonlinear dynamics ==
  data: dist input; x0 input; y output; control input; xk input size=[3,1]; xk1 output size=[3,1]; h parameter
function [y, xk1] = nlrk4(dist, x0, control, xk, h)
    persistent initialized

    if isempty(initialized)
        xk = x0;
        initialized = true;
    end

    function dx = nlf(t,x,u)
    
        % Define constants
        K1 = 10.6608;
        K2 = 0.0487;
        K3 = 0.1031;
        K4 = 404.3827;
        K5 = 0.9442;
        K6 = 1.7125;
        K_tau = 0.0107;
        
        % System equations
        theta = x(1);
        theta_dot = x(2);
        omega = x(3);
        theta_ddot = -K1*sin(theta)-K2*theta_dot-K3*sign(theta_dot)-K_tau*(K4*u-K5*omega-K6*sign(omega));
        omega_dot = K4*u-K5*omega-K6*sign(omega);
        dx = [theta_dot; theta_ddot; omega_dot];
    end

    % Executes one timestep of the RK4 algorithm
    k1 = nlf(0, xk, control);
    k2 = nlf(0 + h/2, xk + h/2*k1, control);
    k3 = nlf(0 + h/2, xk + h/2*k2, control);
    k4 = nlf(0 + h, xk + h*k3, control);
    xk1 = xk + h/6*(k1 + 2*k2 + 2*k3 + k4);


    if dist
        xk1(1)=pi+deg2rad(5);
        xk(1) =pi+deg2rad(5);
    end


    % % Forward Euler
    % xk1 = xk + h*nlf(0, xk, control);
    % Take out states of interest
    y = [xk(1); xk(3)];
end

== matlab function reaction_pendulum_MPC_swing_test/Pendulum nonlinear model2/Nonlinear dynamics ==
  data: H input; x0 input; control input; xp input; xk input size=[3,1]; xk1 output size=[3,1]; h parameter
function xk1   = nlrk4(H, x0, control, xp, xk, h)
    persistent initialized

    if isempty(initialized)
        xk1 = x0;
        theta_dd = 0;
        initialized = true;
        return;
    end

    function dx = nlf(t,x,u,xp,H)
        C = [1,0,0;0,0,1];

        % Define constants
        K1 = 10.6608;
        K2 = 0.0487;
        K3 = 0.1031;
        K4 = 404.3827;
        K5 = 0.9442;
        K6 = 1.7125;
        K_tau = 0.0107;
        
        % System equations
        theta = x(1);
        theta_dot = x(2);
        omega = x(3);
        theta_ddot = -K1*sin(theta)-K2*theta_dot-K3*sign(theta_dot)-K_tau*(K4*u-K5*omega-K6*sign(omega));
        omega_dot = K4*u-K5*omega-K6*sign(omega);
        delta = xp-C*x;
        Linear_term = H*(delta);
        NL_term = [theta_dot; theta_ddot; omega_dot] ;
        dx = NL_term + Linear_term;
    end

    function theta_ddot = theta_ddd(t,x,u,xp,H)
        C = [1,0,0;0,0,1];

        % Define constants
        K1 = 10.6608;
        K2 = 0.0487;
        K3 = 0.1031;
        K4 = 404.3827;
        K5 = 0.9442;
        K6 = 1.7125;
        K_tau = 0.0107;
        
        % System equations
        theta = x(1);
        theta_dot = x(2);
        omega = x(3);
        theta_ddot = -K1*sin(theta)-K2*theta_dot-K3*sign(theta_dot)-K_tau*(K4*u-K5*omega-K6*sign(omega));
    end

    theta_dd = theta_ddd(0, xk, control, xp, H);

    % Executes one timestep of the RK4 algorithm
    k1 = nlf(0, xk, control, xp, H);
    k2 = nlf(0 + h/2, xk + h/2*k1, control, xp + h/2*k1([1,3]), H);
    k3 = nlf(0 + h/2, xk + h/2*k2, control, xp + h/2*k2([1,3]), H);
    k4 = nlf(0 + h, xk + h*k3, control, xp + h*k3([1,3]), H);
    xk1 = xk + h/6*(k1 + 2*k2 + 2*k3 + k4);

    % % Forward Euler
    % xk1 = xk + h*nlf(0, xk, control);
    % Take out states of interest
    % y = [xk(1); xk(3)];
end

== matlab function reaction_pendulum_MPC_swing_test/Pendulum nonlinear model1/Nonlinear dynamics ==
  data: x0 input; control input; xp input; H input; xk input size=[3,1]; xk1 output size=[3,1]; h parameter
function xk1   = nlrk4(x0, control, xp, H, xk, h)
    persistent initialized

    if isempty(initialized)
        xk1 = x0;
        theta_dd = 0;
        initialized = true;
        return;
    end

    function dx = nlf(t,x,u,xp,H)
        C = [1,0,0;0,0,1];

        % Define constants
        K1 = 10.6608;
        K2 = 0.0487;
        K3 = 0.1031;
        K4 = 404.3827;
        K5 = 0.9442;
        K6 = 1.7125;
        K_tau = 0.0107;
        
        % System equations
        theta = x(1);
        theta_dot = x(2);
        omega = x(3);
        theta_ddot = -K1*sin(theta)-K2*theta_dot-K3*sign(theta_dot)-K_tau*(K4*u-K5*omega-K6*sign(omega));
        omega_dot = K4*u-K5*omega-K6*sign(omega);
        delta = xp-C*x;
        Linear_term = H*(delta);
        NL_term = [theta_dot; theta_ddot; omega_dot] ;
        dx = NL_term + Linear_term;
    end

    function theta_ddot = theta_ddd(t,x,u,xp,H)
        C = [1,0,0;0,0,1];

        % Define constants
        K1 = 10.6608;
        K2 = 0.0487;
        K3 = 0.1031;
        K4 = 404.3827;
        K5 = 0.9442;
        K6 = 1.7125;
        K_tau = 0.0107;
        
        % System equations
        theta = x(1);
        theta_dot = x(2);
        omega = x(3);
        theta_ddot = -K1*sin(theta)-K2*theta_dot-K3*sign(theta_dot)-K_tau*(K4*u-K5*omega-K6*sign(omega));
    end

    theta_dd = theta_ddd(0, xk, control, xp, H);

    % Executes one timestep of the RK4 algorithm
    k1 = nlf(0, xk, control, xp, H);
    k2 = nlf(0 + h/2, xk + h/2*k1, control, xp + h/2*k1([1,3]), H);
    k3 = nlf(0 + h/2, xk + h/2*k2, control, xp + h/2*k2([1,3]), H);
    k4 = nlf(0 + h, xk + h*k3, control, xp + h*k3([1,3]), H);
    xk1 = xk + h/6*(k1 + 2*k2 + 2*k3 + k4);

    % % Forward Euler
    % xk1 = xk + h*nlf(0, xk, control);
    % Take out states of interest
    % y = [xk(1); xk(3)];
end
